simulink model "FDM"  (R2018a)
settings: Solver=VariableStepAuto  StartTime=0.0  StopTime=10.0  RelTol=1e-3
settings Model: Creator=Sohan  LastModifiedBy=Sohan

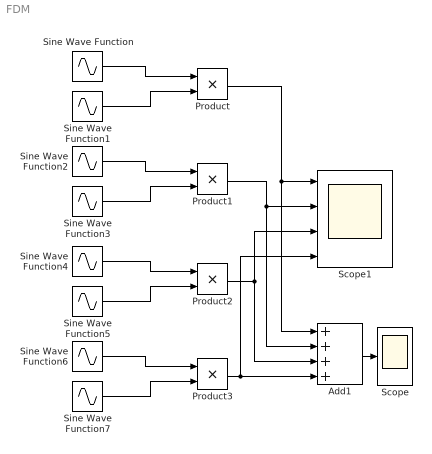
== system FDM ==
  Add1 : Sum  Inputs=++++
  Product{,1..3} (4 alike) : Product
  Scope : Scope
  Scope1 : Scope  NumInputPorts=4
  Sine Wave Function : Sin  Amplitude=0.5  SampleTime=0
  Sine Wave Function1 : Sin  Frequency=3  SampleTime=0
  Sine Wave Function2 : Sin  Amplitude=0.5  Frequency=2  SampleTime=0
  Sine Wave Function3 : Sin  Frequency=4  SampleTime=0
  Sine Wave Function4 : Sin  Amplitude=0.5  Frequency=3  SampleTime=0
  Sine Wave Function5 : Sin  Frequency=5  Samples=5  SampleTime=0
  Sine Wave Function6 : Sin  Amplitude=0.5  Frequency=6  Samples=6  SampleTime=0
  Sine Wave Function7 : Sin  Frequency=7  SampleTime=0
  wires:
  Sine Wave Function/1 -> Product/1
  Sine Wave Function1/1 -> Product/2
  Sine Wave Function2/1 -> Product1/1
  Sine Wave Function3/1 -> Product1/2
  Sine Wave Function4/1 -> Product2/1
  Sine Wave Function5/1 -> Product2/2
  Sine Wave Function6/1 -> Product3/1
  Sine Wave Function7/1 -> Product3/2
  Product/1 -> Add1/1, Scope1/1
  Product1/1 -> Scope1/2, Add1/2
  Product2/1 -> Scope1/3, Add1/3
  Product3/1 -> Scope1/4, Add1/4
  Add1/1 -> Scope/1
